simulink model "test_var"  (R2023b)
settings: Solver=VariableStepAuto  StartTime=0.0  StopTime=1  RelTol=1e-3
values from neighbouring files (symbols this model uses):
  idx_rand = randi([1, 2000], 1, 1)    [code_lsandtrain.m]
  in = data.in    [code_lsandtrain.m]
  out = data.out    [code_lsandtrain.m]
settings Model: Creator=Jhchen  LastModifiedBy=Jhchen
settings DataIOCC: ReturnWorkspaceOutputs=off

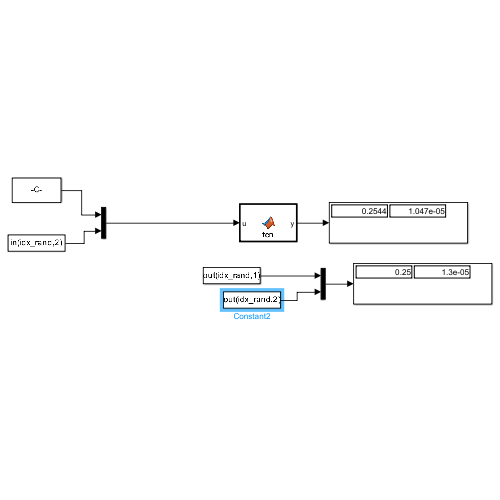
[thumbnail: Simulink's stored preview of the top-level diagram]
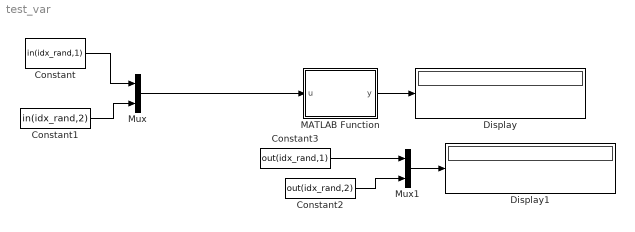
== system test_var ==
  Constant : Constant  Value=in(idx_rand,1)
  Constant1 : Constant  Value=in(idx_rand,2)
  Constant2 : Constant  Value=out(idx_rand,2)
  Constant3 : Constant  Value=out(idx_rand,1)
  Display : Display
  Display1 : Display
  MATLAB Function : MATLAB Function  TreatAsAtomicUnit=on
  Mux : Mux  Inputs=2
  Mux1 : Mux  Inputs=2
  wires:
  Constant/1 -> Mux/1
  Constant1/1 -> Mux/2
  MATLAB Function/1(y) -> Display/1
  Mux/1 -> MATLAB Function/1(u)
  Constant3/1 -> Mux1/1
  Constant2/1 -> Mux1/2
  Mux1/1 -> Display1/1

== matlab function test_var/MATLAB Function ==
  data: u input; y output
function y = fcn(u)

y = predict(u);
